simulink model "Demo_4481"  (R2021a)
settings: Solver=VariableStepAuto  StartTime=0.0  StopTime=10.0  RelTol=1e-3
settings Model: Creator=Willi  LastModifiedBy=Willi

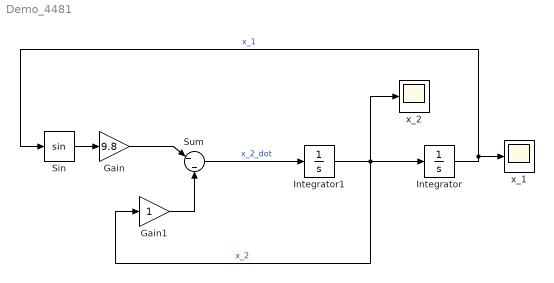
== system Demo_4481 ==
  Gain : Gain  Gain=9.8
  Gain1 : Gain
  Integrator : Integrator  InitialCondition=1
  Integrator1 : Integrator  InitialCondition=1
  Sin : Trigonometry
  Sum : Sum  Inputs=|-|-
  x_1 : Scope
  x_2 : Scope
  wires:
  Sin/1 -> Gain/1
  Gain/1 -> Sum/1
  Gain1/1 -> Sum/2
  Sum/1 -> Integrator1/1  "x_2_dot"
  Integrator/1 -> x_1/1, Sin/1  "x_1"
  Integrator1/1 -> x_2/1, Integrator/1, Gain1/1  "x_2"
